simulink model "untitled1"  (R2020a)
settings: Solver=VariableStepAuto  StartTime=0.0  StopTime=10.0  MaxStep=0.01  RelTol=1e-3
InitFcn:
  | F =50;
  | m = 2;
  | k = 0.1;
  | b =10;
values from neighbouring files (symbols this model uses):
  c = input('c degerini giriniz:')    [kokbul.m]
undefined symbols (not defined in the file or in its folder): l, r
settings Model: Creator=muham  LastModifiedBy=muham

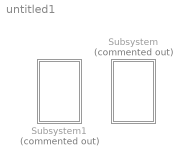
== system untitled1 ==
  Subsystem : Subsystem  Commented=on
  Subsystem1 : Subsystem  Commented=on

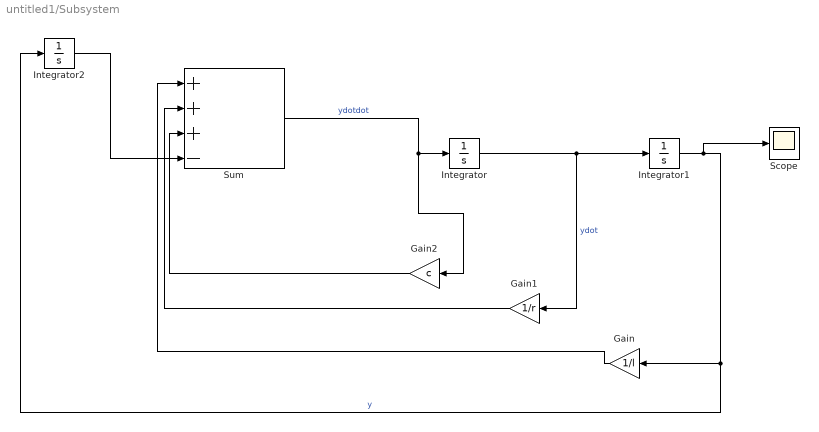
== system untitled1/Subsystem ==
  Gain : Gain  Gain=1/l
  Gain1 : Gain  Gain=1/r
  Gain2 : Gain  Gain=c
  Integrator : Integrator
  Integrator1 : Integrator
  Integrator2 : Integrator
  Scope : Scope
  Sum : Sum  Inputs=|+++-
  wires:
  Integrator/1 -> Gain1/1, Integrator1/1  "ydot"
  Integrator1/1 -> Integrator2/1, Gain/1, Scope/1  "y"
  Gain1/1 -> Sum/2
  Integrator2/1 -> Sum/4
  Gain/1 -> Sum/1
  Sum/1 -> Gain2/1, Integrator/1  "ydotdot"
  Gain2/1 -> Sum/3

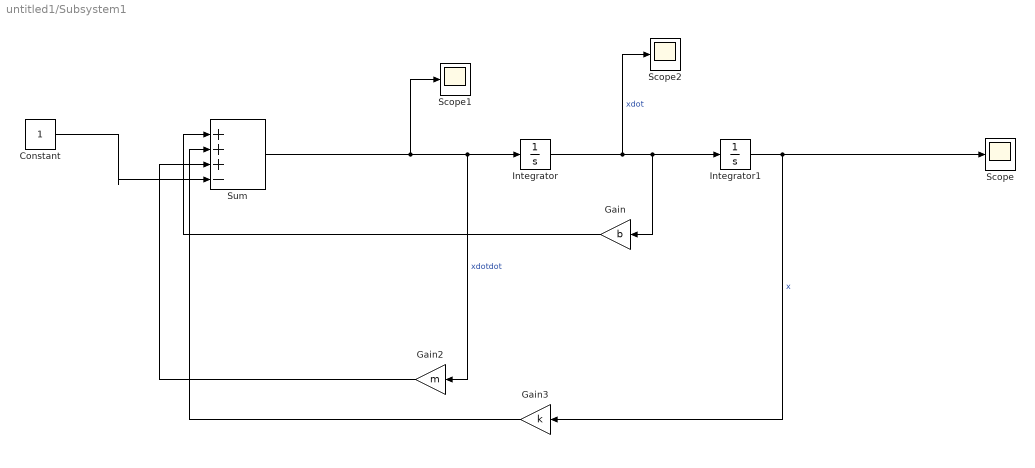
== system untitled1/Subsystem1 ==
  Constant : Constant
  Gain : Gain  Gain=b
  Gain2 : Gain  Gain=m
  Gain3 : Gain  Gain=k
  Integrator : Integrator
  Integrator1 : Integrator
  Scope : Scope
  Scope1 : Scope
  Scope2 : Scope
  Sum : Sum  Inputs=|+++-
  wires:
  Constant/1 -> Sum/4
  Gain/1 -> Sum/1
  Sum/1 -> Scope1/1, Gain2/1, Integrator/1  "xdotdot"
  Integrator1/1 -> Scope/1, Gain3/1  "x"
  Integrator/1 -> Scope2/1, Gain/1, Integrator1/1  "xdot"
  Gain3/1 -> Sum/2
  Gain2/1 -> Sum/3
